simulink model "PID_ControlLoop"  (R2018a)
settings: Solver=VariableStepAuto  StartTime=0.0  StopTime=10.0  RelTol=1e-3
settings Model: Creator=rahul  LastModifiedBy=rahul

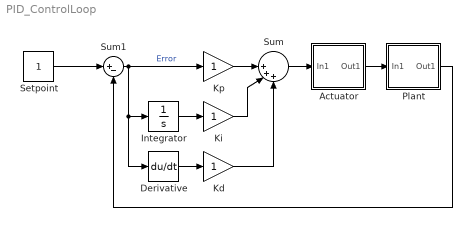
== system PID_ControlLoop ==
  Actuator : Subsystem
  Derivative : Derivative
  Integrator : Integrator
  Kd : Gain
  Ki : Gain
  Kp : Gain
  Plant : Subsystem
  Setpoint : Constant
  Sum : Sum  Inputs=||+++
  Sum1 : Sum  Inputs=|+-
  wires:
  Derivative/1 -> Kd/1
  Integrator/1 -> Ki/1
  Kp/1 -> Sum/1
  Kd/1 -> Sum/3
  Sum1/1 -> Derivative/1, Integrator/1, Kp/1  "Error"
  Setpoint/1 -> Sum1/1
  Sum/1 -> Actuator/1(In1)
  Ki/1 -> Sum/2
  Actuator/1(Out1) -> Plant/1(In1)
  Plant/1(Out1) -> Sum1/2

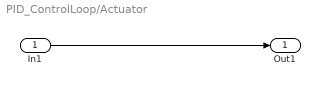
== system PID_ControlLoop/Actuator ==
  In1 : Inport
  Out1 : Outport
  wires:
  In1/1 -> Out1/1

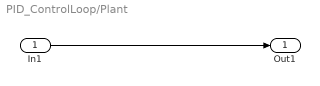
== system PID_ControlLoop/Plant ==
  In1 : Inport
  Out1 : Outport
  wires:
  In1/1 -> Out1/1
